simulink model "STEVE_Simulation"  (R2025b)
settings: Solver=ode8  StartTime=0  StopTime=300  FixedStep=0.0001  MaxStep=0.0001  RelTol=1e-3
model workspace (MAT data in the model file):
  op_trim1 : opcond.OperatingReport (value not decoded)
undefined symbols (not defined in the file): a_gyro_fast, Actuators, AeroData, b_gyro_fast, C_inner_launch_d_Kd, C_inner_launch_d_Ki, C_inner_launch_d_Kp, C_inner_maxQ_d_Kd, C_inner_maxQ_d_Ki, C_inner_maxQ_d_Kp, C_inner_maxQ_d_Tf, C_outer_launch_d_Kd, C_outer_launch_d_Ki, C_outer_launch_d_Kp, C_outer_launch_d_N, C_outer_maxQ_d_Kd, C_outer_maxQ_d_Ki, C_outer_maxQ_d_Kp, dspblkCoreblockFVToolHelper, F, fractalcoef, fs_filter, fs_gyro, gcbh, Initial, K_gains, Light, max_q_margin, MIL, PrelookupData, Ref_Area, rocket_length, RocketAeroPhysical, time_vector, timeStep, Ts_inner, Ts_outer, wn_ramp
libraries: simulink x14, simulink_extras x11, slpidlib x10, aerolibwind2 x3, aerolibasang x3, aerolibtransform2 x2, aerolibatmos2 x1, sensorgpslib x1, mspsensorlib x1, aerolibconvert2 x1, aerolibactuator x1
(part 3 of 3)

== system STEVE_Simulation/STeVe System Model/Vehicle Dynamics/Aerodynamics/Force Calculations ==
  Ref Area : Inport
  CN : Inport  Port=2
  CA : Inport  Port=3
  CP : Inport  Port=4
  qbar : Inport  Port=5
  CG : Inport  Port=6
  omega : Inport  Port=7
  V : Inport  Port=8
  CMq : Inport  Port=9
  (1 to force stable) : Gain  Gain=-1
  Constant : Constant  Value=rocket_length
  Constant1 : Constant  Value=Ref_Area
  MATLAB Function : MATLAB Function  TreatAsAtomicUnit=on
  Multiply : Gain  Gain=-1
  Multiply1 : Gain
  Multiply2 : Gain  Gain=-1
  Product : Product  Inputs=***
  Product1 : Product  Inputs=***
  Product2 : Product
  Selector : Selector  InputPortWidth=3  IndexOptions=Index vector (dialog)  Indices=2  OutputSizes=1
  Sum : Sum  Inputs=|-+
  Sum1 : Sum  Inputs=|-+
  Sum3 : Sum  Inputs=|++
  qbar1 : InportShadow  Port=5
  "Axial Force, Body" : Outport
  "Normal Force, Body" : Outport  Port=2
  "Pitching Momen, Body" : Outport  Port=3
  tag scope: L_ref=global
  wires:
  Product/1 -> "Axial Force, Body"/1  "Axial Force Aero"
  CA/1 -> Multiply/1
  qbar/1 -> Product/3, Product1/2  "q_bar"
  Ref Area/1 -> Product/2, Product1/1  "ref_area"
  Multiply/1 -> Product/1
  Multiply2/1 -> Product1/3  "CN"
  CP/1 -> Sum1/1  "CP (from nose)"
  Sum1/1 -> (1 to force stable)/1, [L_ref]  "Lref"
  Product2/1 -> Sum3/1  "Moment no damp"
  Sum3/1 -> Multiply1/1  "Total"
  Sum/1 -> Sum1/2  "CG (from nose)"
  Constant/1 -> MATLAB Function/1(L), Sum/2
  Multiply1/1 -> "Pitching Momen, Body"/1
  Product1/1 -> Product2/1, "Normal Force, Body"/1  "Normal Force Aero"
  V/1 -> MATLAB Function/4(V)  "V wind"
  omega/1 -> Selector/1
  Selector/1 -> MATLAB Function/3(q)  "q_pitch"
  qbar1/1 -> MATLAB Function/5(q_bar)  "q_bar"
  CG/1 -> Sum/1  "CG (from aft)"
  (1 to force stable)/1 -> Product2/2
  Constant1/1 -> MATLAB Function/6(S)
  MATLAB Function/1(dampingMoment) -> Sum3/2  "damping Moment"
  CMq/1 -> MATLAB Function/2(Cmq_derivative)
  CN/1 -> Multiply2/1  "CN"

== system STEVE_Simulation/STeVe System Model/Vehicle Dynamics/Propulsion F,M/Subsystem ==
  Thrust : Inport
  Nozzle Angle : Inport  Port=2
  CG : Inport  Port=3
  Cos : Trigonometry  Operator=cos
  Product : Product
  Product1 : Product  OutDataTypeStr=double
  Product2 : Product
  Sin : Trigonometry
  Ft_x_b : Outport
  Ft_z_b : Outport  Port=2
  M_y_b : Outport  Port=3
  wires:
  Nozzle Angle/1 -> Sin/1, Cos/1
  Thrust/1 -> Product1/1, Product/1
  Product/1 -> Ft_x_b/1
  Cos/1 -> Product/2
  Product1/1 -> Product2/1, Ft_z_b/1
  Sin/1 -> Product1/2
  Product2/1 -> M_y_b/1
  CG/1 -> Product2/2

== system STEVE_Simulation/STeVe System Model/Vehicle Dynamics/Time Varying Parameters/TimeToIndex ==
  t : Inport
  Add Constant : Bias  Bias=1  SaturateOnIntegerOverflow=off
  Constant : Constant  Value=timeStep
  Product : Product  Inputs=*/
  Index : Outport
  wires:
  t/1 -> Product/1
  Constant/1 -> Product/2
  Product/1 -> Add Constant/1
  Add Constant/1 -> Index/1

== system STEVE_Simulation/STeVe System Model/Vehicle Dynamics/3DOF to 6DOF/3DOF to 6DOF/calc alpha_dot ==
  "alpha, beta" : Inport
  Ab : Inport  Port=2
  Vw : Inport  Port=3
  "Add epsilon to avoid division by 0 " : Bias  Bias=1*10^-8  SaturateOnIntegerOverflow=off
  Direction Cosine Matrix Body to Wind : aerolibtransform2/Direction Cosine Matrix Body to Wind
  Matrix Multiply : Product  Multiplication=Matrix(*)
  Product : Product  Inputs=*/
  Selector : Selector  IndexMode=Zero-based  InputPortWidth=3  IndexOptions=Index vector (dialog)  Indices=2  OutputSizes=1
  Selector1 : Selector  IndexMode=Zero-based  InputPortWidth=3  IndexOptions=Index vector (dialog)  Indices=0  OutputSizes=1
  alpha_dot : Outport
  wires:
  "alpha, beta"/1 -> Direction Cosine Matrix Body to Wind/1
  Direction Cosine Matrix Body to Wind/1 -> Matrix Multiply/1
  Ab/1 -> Matrix Multiply/2
  Matrix Multiply/1 -> Selector/1
  Vw/1 -> Selector1/1
  Selector/1 -> Product/1
  Selector1/1 -> "Add epsilon to avoid division by 0 "/1
  Product/1 -> alpha_dot/1
  "Add epsilon to avoid division by 0 "/1 -> Product/2

== matlab function STEVE_Simulation/STeVe System Model/Vehicle Dynamics/RocketEngineActuators/MATLAB Function ==
  data: altitude input; thrust output
function thrust = fcn(altitude)

thrust = -3.75507*10^(-2)*altitude + 2.76476*10^(4);

== matlab function STEVE_Simulation/Environment/g(h) ==
  data: h input; g output
function g = fcn(h)
G = 6.67430*10^(-11);
M = 5.9722*10^(24);
R_e = 6.371*10^(6);

g = (G * M)/(R_e + h)^2;

== matlab function STEVE_Simulation/STeVe System Model/Control System/Classical Upgraded/MATLAB Function1 ==
  data: qbar input; blended_output output; qbar_max input; output_launch input; output_maxQ input
function blended_output = blend_controllers(qbar, qbar_max, output_launch, output_maxQ)
% blend_controllers blends two controller outputs based on qbar
% Inputs:
%   qbar        - current dynamic pressure
%   qbar_max    - maximum dynamic pressure reference
%   output_launch - controller output at launch
%   output_maxQ   - controller output at max Q
%
% Output:
%   blended_output - weighted/blended controller output

    w = qbar / qbar_max;
    if w < 0
        w = 0;
    elseif w > 1
        w = 1;
    end
    blended_output = (1 - w) * output_launch + w * output_maxQ;
end

== matlab function STEVE_Simulation/STeVe System Model/Vehicle Dynamics/Aerodynamics/Force Calculations/MATLAB Function ==
  data: L input; dampingMoment output; Cmq_derivative input; q input; V input; q_bar input; S input; Cm_damping_coeff output
function [dampingMoment, Cm_damping_coeff] = calculateDampingMoment(L, Cmq_derivative, q, V, q_bar, S)
% Calculates the dimensional pitch damping moment from the dimensionless Cmq derivative.
%
% Inputs:
%   L:              Reference length (m)
%   Cmq_derivative: The dimensionless pitch damping derivative (from lookup or approximation)
%   q:              Pitch angular velocity (rad/s)
%   V:              Vehicle velocity (m/s)
%   q_bar:          Dynamic pressure (Pa)
%   S:              Reference area (m^2)
%
% Outputs:
%   dampingMoment:      The final physical damping moment (N*m)
%   Cm_damping_coeff:   The intermediate dimensionless damping moment coefficient

    % Handle the V=0 case to prevent division by zero
    if V == 0
        non_dim_pitch_rate = 0;
    else
        % Calculate the non-dimensional pitch rate (q_hat)
        non_dim_pitch_rate = (q * L) / (2 * V);
    end

    % Calculate the total damping moment coefficient
    Cm_damping_coeff = Cmq_derivative * non_dim_pitch_rate;

    % Convert the coefficient to a physical moment
    dampingMoment = Cm_damping_coeff * q_bar * S * L;

end

== matlab function STEVE_Simulation/STeVe System Model/Control System/Classical Upgraded/MATLAB Function ==
  data: total_aero_moment input; delta_ff output; T input; L_arm input
function delta_ff = feedforward_calculator(total_aero_moment, T, L_arm)
% This function calculates the feedforward TVC angle (delta_ff) required
% to counteract the aerodynamic moments acting on the rocket.

% --- SOLUTION: Initialize the output variable explicitly ---
% This tells the Simulink Coder that delta_ff is always a 1x1 double.
delta_ff = 0.0;

% --- Safety Check: Prevent division by zero if thrust is negligible ---
if T < 1.0 || abs(T * L_arm) < 1e-6
    % We've already initialized delta_ff to 0, so we can just exit.
    return;
end

% --- Calculate the TVC command to counteract this moment ---
% The required control moment is equal and opposite to the aero moment.
required_tvc_moment = -total_aero_moment*1;

% Convert the required moment into a nozzle angle command.
% The double() cast prevents data type mismatch errors.
delta_ff = double(required_tvc_moment / (T * L_arm));

end

== matlab function STEVE_Simulation/STeVe System Model/Control System/LQR1/MATLAB Function ==
  data: total_aero_moment input; delta_ff output; T input; L_arm input
function delta_ff = feedforward_calculator(total_aero_moment, T, L_arm)
% This function calculates the feedforward TVC angle (delta_ff) required
% to counteract the aerodynamic moments acting on the rocket.

% --- SOLUTION: Initialize the output variable explicitly ---
% This tells the Simulink Coder that delta_ff is always a 1x1 double.
delta_ff = 0.0;

% --- Safety Check: Prevent division by zero if thrust is negligible ---
if T < 1.0 || abs(T * L_arm) < 1e-6
    % We've already initialized delta_ff to 0, so we can just exit.
    return;
end

% --- Calculate the TVC command to counteract this moment ---
% The required control moment is equal and opposite to the aero moment.
required_tvc_moment = -total_aero_moment;

% Convert the required moment into a nozzle angle command.
% The double() cast prevents data type mismatch errors.
delta_ff = double(required_tvc_moment / (T * L_arm));

end

== matlab function STEVE_Simulation/STeVe System Model/Control System/Classical Upgraded2/MATLAB Function ==
  data: total_aero_moment input; delta_ff output; T input; L_arm input
function delta_ff = feedforward_calculator(total_aero_moment, T, L_arm)
% This function calculates the feedforward TVC angle (delta_ff) required
% to counteract the aerodynamic moments acting on the rocket.

% --- SOLUTION: Initialize the output variable explicitly ---
% This tells the Simulink Coder that delta_ff is always a 1x1 double.
delta_ff = 0.0;

% --- Safety Check: Prevent division by zero if thrust is negligible ---
if T < 1.0 || abs(T * L_arm) < 1e-6
    % We've already initialized delta_ff to 0, so we can just exit.
    return;
end

% --- Calculate the TVC command to counteract this moment ---
% The required control moment is equal and opposite to the aero moment.
required_tvc_moment = -total_aero_moment*1;

% Convert the required moment into a nozzle angle command.
% The double() cast prevents data type mismatch errors.
delta_ff = double(required_tvc_moment / (T * L_arm));

end

== matlab function STEVE_Simulation/STeVe System Model/Control System/Classical Upgraded2/MATLAB Function1 ==
  data: qbar input; blended_output output; qbar_max input; output_launch input; output_maxQ input
function blended_output = blend_controllers(qbar, qbar_max, output_launch, output_maxQ)
% blend_controllers blends two controller outputs based on qbar
% Inputs:
%   qbar        - current dynamic pressure
%   qbar_max    - maximum dynamic pressure reference
%   output_launch - controller output at launch
%   output_maxQ   - controller output at max Q
%
% Output:
%   blended_output - weighted/blended controller output

    w = qbar / qbar_max;
    if w < 0
        w = 0;
    elseif w > 1
        w = 1;
    end
    blended_output = (1 - w) * output_launch + w * output_maxQ;
end
